simulink model "lotkavolterra-simulink"  (R2022a)
settings: Solver=VariableStepAuto  StartTime=0.0  StopTime=20  FixedStep=0.001  RelTol=1e-3
settings Model: Creator=barrt  LastModifiedBy=barrt

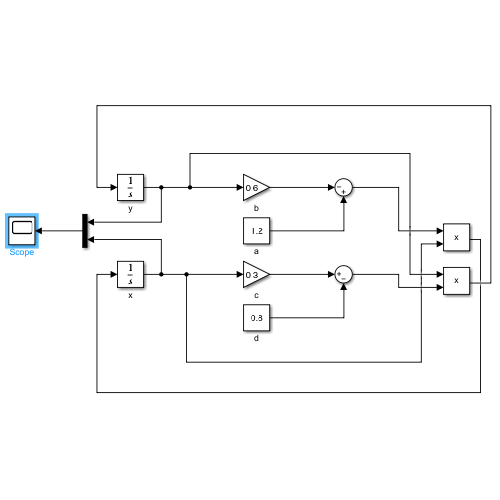
[thumbnail: Simulink's stored preview of the top-level diagram]
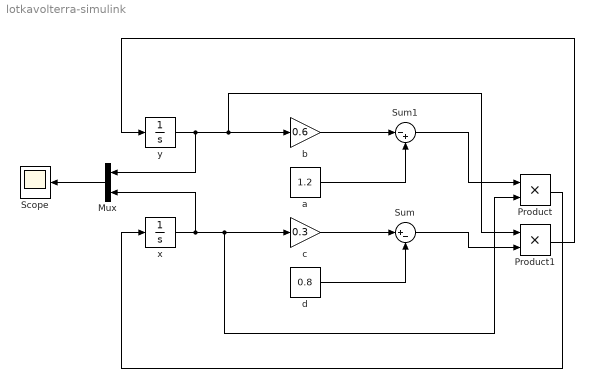
== system lotkavolterra-simulink ==
  Mux : Mux  Inputs=2
  Product : Product
  Product1 : Product
  Scope : Scope
  Sum : Sum  Inputs=|+-
  Sum1 : Sum  Inputs=|-+
  a : Constant  Value=1.2
  b : Gain  Gain=0.6
  c : Gain  Gain=0.3
  d : Constant  Value=0.8
  x : Integrator  InitialCondition=2
  y : Integrator  InitialCondition=1
  wires:
  y/1 -> Mux/1, Product1/1, b/1
  x/1 -> Mux/2, Product/2, c/1
  b/1 -> Sum1/1
  a/1 -> Sum1/2
  c/1 -> Sum/1
  d/1 -> Sum/2
  Sum/1 -> Product1/2
  Sum1/1 -> Product/1
  Product1/1 -> y/1
  Product/1 -> x/1
  Mux/1 -> Scope/1
